simulink model "sis_massa_molla"  (R2020b)
settings: Solver=VariableStepAuto  StartTime=0.0  StopTime=T  MaxStep=0.1  RelTol=1e-3
values from neighbouring files (symbols this model uses):
  A = [0 1;-k/m -b/m]    [risposta_gradino.m]
  B = [0; 1/m]    [risposta_gradino.m]
  C = [1 0]    [risposta_gradino.m]
  D = 0    [risposta_gradino.m]
  x0 = [1 ; 0]    [risposta_gradino.m]
settings Model: Creator=Lenovo  LastModifiedBy=Lenovo

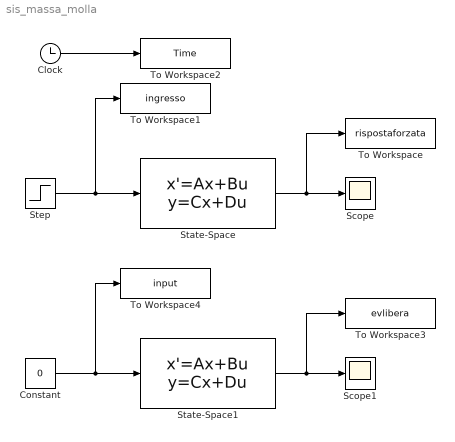
== system sis_massa_molla ==
  Clock : Clock
  Constant : Constant  Value=0
  Scope : Scope
  Scope1 : Scope
  State-Space : StateSpace  A=A  B=B  C=C  D=D  InitialCondition=x0
  State-Space1 : StateSpace  A=A  B=B  C=C  D=D  InitialCondition=x0
  Step : Step  SampleTime=0
  To Workspace : ToWorkspace  VariableName=rispostaforzata  SampleTime=-1
  To Workspace1 : ToWorkspace  VariableName=ingresso  SampleTime=-1
  To Workspace2 : ToWorkspace  VariableName=Time  SampleTime=-1
  To Workspace3 : ToWorkspace  VariableName=evlibera  SampleTime=-1
  To Workspace4 : ToWorkspace  VariableName=input  SampleTime=-1
  wires:
  State-Space/1 -> To Workspace/1, Scope/1
  Clock/1 -> To Workspace2/1
  Step/1 -> To Workspace1/1, State-Space/1
  Constant/1 -> To Workspace4/1, State-Space1/1
  State-Space1/1 -> To Workspace3/1, Scope1/1
